simulink model "es1_catena_aperta_2"  (R2014a)
settings: Solver=ode45  StartTime=0.0  StopTime=20.0  RelTol=1e-3
values from neighbouring files (symbols this model uses):
  beta = 0.02    [es1.m]
  Ka = 10    [es1.m]
  Km = 0.5    [es1.m]
  Ra = 1    [es1.m]
libraries: cstblocks x2
settings Model: Creator=HP  LastModifiedBy=HP
settings DataIOCC: InspectSignalLogs=on

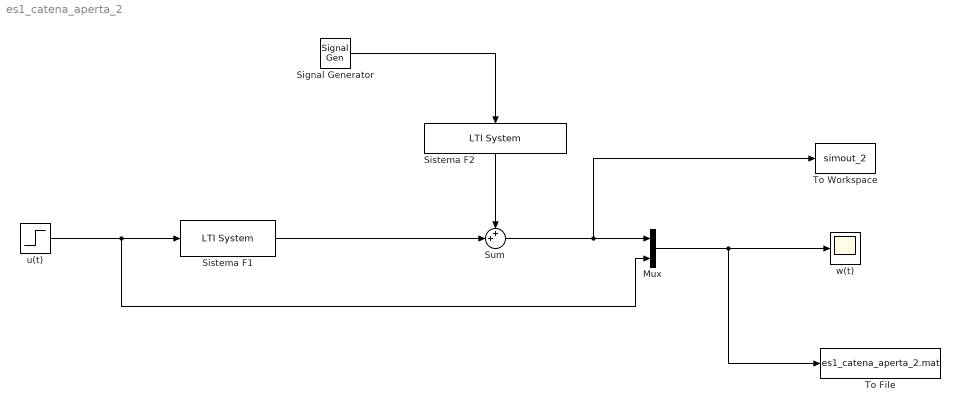
== system es1_catena_aperta_2 ==
  Mux : Mux  Inputs=2
  Signal Generator : SignalGenerator  WaveForm=square  Amplitude=0.05  Frequency=0.1
  Sistema F1 : cstblocks/LTI System  sys=F1  IC=[]
  Sistema F2 : cstblocks/LTI System  sys=F2  IC=[]
  Sum : Sum  Inputs=++|
  To File : ToFile  Filename=es1_catena_aperta_2.mat  MatrixName=output_2  SaveFormat=Timeseries
  To Workspace : ToWorkspace  VariableName=simout_2  SaveFormat=Timeseries  SampleTime=-1
  u(t) : Step  Time=0  After=((Ka * Km) / (beta * Ra + Km*Km))^-1  SampleTime=0
  w(t) : Scope
      settings: MaxDataPoints=100000
  wires:
  u(t)/1 -> Mux/2, Sistema F1/1
  Sistema F2/1 -> Sum/1
  Sistema F1/1 -> Sum/2
  Sum/1 -> To Workspace/1, Mux/1
  Mux/1 -> To File/1, w(t)/1
  Signal Generator/1 -> Sistema F2/1
